simulink model "VDCHyd2022a"  (R2022a)
settings: Solver=daessc  StartTime=0.0  StopTime=simulationEndTime  FixedStep=0.001  RelTol=1e-2
values from neighbouring files (symbols this model uses):
  aux = thetaXrLB(i)    [initInertiaUpdate.m]
  Bc1_V = [0;0;0;0;0;0]    [InitializeSimulationParameters.m]
  Bc1_Vr = [0;0;0;0;0;0]    [InitializeSimulationParameters.m]
  D22Fr = [0;0;0;0;0;0]    [InitializeSimulationParameters.m]
  filtDF = init2ndOrderLowPassFilter(filtDF.cutOffFrequency,1,controller.dT)    [initializeLowPassFilters.m]
  filtDV = init2ndOrderLowPassFilter(filtDV.cutOffFrequency,1,controller.dT)    [initializeLowPassFilters.m]
  filtEnc = init2ndOrderLowPassFilter(filtEnc.cutOffFrequency,1,controller.dT)    [initializeLowPassFilters.m]
  filtPres = init2ndOrderLowPassFilter(filtPres.cutOffFrequency,1,controller.dT)    [initializeLowPassFilters.m]
  MODE = 1    [RUN_ME.m]
  s = tf('s')    [init2ndOrderLowPassFilter.m]
undefined symbols (not defined in the file or in its folder): B11_r_B11Tc1, B11_V, B11_Vr, B11Ftot_r, B12_r_B12Tc2, B12_Rot_Tc2, B12_U_Tc2, B12_V, B12_Vr, B12Ftot_r, B31_r_B31B41, B31_V, B31_Vr, B31FTot_r, B32_r_B32B42, B32_Rot_B42, B32_U_B42, B32_V, B32_Vr, B32FTot_r, B41_r_B41Tc1, B41_V, B41_Vr, B41FTot_r, B42_r_B42Tc2, B42_Rot_Tc2, B42_U_Tc2, B42_V, B42_Vr, B42FTot_r, B52_r_B52P32, B52_Rot_P32, B52_U_P32, B52_V, B52_Vr, B52Ftot_r, Bc1_r_Bc1B11, Bc1_r_Bc1B31, Bc1FTot_r, Bc2_r_Bc2B12, Bc2_r_Bc2B32, Bc2_Rot_B12, Bc2_Rot_B32, Bc2_U_B12, Bc2_U_B32, Bc2_V, Bc2_Vr, Bc2Tot_r, controller, cyl1, cyl2, cylT2, D22_V, D22_Vr, DiscIntNeverNeededParam, dq1, dq11, dq11r, dq12, dq12r ... (+119)
libraries: sm_lib x34, nesl_utility x15, simulink x11, dspinverses x1
(part 10 of 12)

== system VDCHyd2022a/sbVDCController/sbFormTotalRequiredForces/sbTotalRequiredForcesRS2/sbFilteredVelocityDerivativeB32/sbLowPassFilter6 ==
  dV : Inport
  Delay : Delay  InitialConditionSource=Input port  SampleTime=filtDV.dT
      settings: InputPortMap=u0,p4
  Delay1 : Delay  DelayLength=1  InitialConditionSource=Input port  SampleTime=filtDV.dT
      settings: InputPortMap=u0,p4
  Delay2 : Delay  DelayLength=0  InitialConditionSource=Input port  SampleTime=filtDV.dT
      settings: InputPortMap=u0,p4
  Delay3 : Delay  InitialConditionSource=Input port  SampleTime=filtDV.dT
      settings: InputPortMap=u0,p4
  Delay4 : Delay  DelayLength=1  InitialConditionSource=Input port  SampleTime=filtDV.dT
      settings: InputPortMap=u0,p4
  Gain : Gain  Gain=filtDV.a0
  Gain1 : Gain  Gain=filtDV.b1
  Gain2 : Gain  Gain=filtDV.b2
  Gain3 : Gain  Gain=filtDV.b0
  Gain4 : Gain  Gain=filtDV.a1
  Sum : Sum  Inputs=|--+++
  dVFilt : Outport
  wires:
  Delay3/1 -> Gain3/1
  Gain/1 -> Sum/2
  Gain1/1 -> Sum/4
  dV/1 -> Delay/2, Delay4/2, Delay1/2, Delay3/1, Delay3/2, Delay1/1, Delay2/2, Delay2/1  "dV"
  Sum/1 -> Delay/1, Delay4/1, dVFilt/1  "dVFilt"
  Gain4/1 -> Sum/1
  Delay2/1 -> Gain2/1
  Delay1/1 -> Gain1/1
  Delay/1 -> Gain/1
  Delay4/1 -> Gain4/1
  Gain2/1 -> Sum/3
  Gain3/1 -> Sum/5

== system VDCHyd2022a/sbVDCController/sbFormTotalRequiredForces/sbTotalRequiredForcesRS2/sbFilteredVelocityDerivativeB42/sbDiscreteDerivative1 ==
  u : Inport
  Add : Sum  Inputs=-+
  Gain6 : Gain  Gain=1/(2*controller.dT)
  Integer Delay : Delay  InitialConditionSource=Input port  InitialCondition=0  SampleTime=controller.dT
      settings: InputPortMap=u0,p4
  du/dt : Outport  PortDimensions=1
  wires:
  Add/1 -> Gain6/1
  u/1 -> Integer Delay/1, Integer Delay/2, Add/2
  Integer Delay/1 -> Add/1
  Gain6/1 -> du/dt/1

== system VDCHyd2022a/sbVDCController/sbFormTotalRequiredForces/sbTotalRequiredForcesRS2/sbFilteredVelocityDerivativeB42/sbDiscreteDerivative2 ==
  u : Inport
  Add : Sum  Inputs=-+
  Gain6 : Gain  Gain=1/(2*controller.dT)
  Integer Delay : Delay  InitialConditionSource=Input port  InitialCondition=0  SampleTime=controller.dT
      settings: InputPortMap=u0,p4
  du/dt : Outport  PortDimensions=1
  wires:
  u/1 -> Integer Delay/1, Integer Delay/2, Add/2
  Integer Delay/1 -> Add/1
  Add/1 -> Gain6/1
  Gain6/1 -> du/dt/1

== system VDCHyd2022a/sbVDCController/sbFormTotalRequiredForces/sbTotalRequiredForcesRS2/sbFilteredVelocityDerivativeB42/sbDiscreteDerivative3 ==
  u : Inport
  Add : Sum  Inputs=-+
  Gain6 : Gain  Gain=1/(2*controller.dT)
  Integer Delay : Delay  InitialConditionSource=Input port  InitialCondition=0  SampleTime=controller.dT
      settings: InputPortMap=u0,p4
  du/dt : Outport  PortDimensions=1
  wires:
  Add/1 -> Gain6/1
  Integer Delay/1 -> Add/1
  u/1 -> Integer Delay/1, Integer Delay/2, Add/2
  Gain6/1 -> du/dt/1

== system VDCHyd2022a/sbVDCController/sbFormTotalRequiredForces/sbTotalRequiredForcesRS2/sbFilteredVelocityDerivativeB42/sbDiscreteDerivative4 ==
  u : Inport
  Add : Sum  Inputs=-+
  Gain6 : Gain  Gain=1/(2*controller.dT)
  Integer Delay : Delay  InitialConditionSource=Input port  InitialCondition=0  SampleTime=controller.dT
      settings: InputPortMap=u0,p4
  du/dt : Outport  PortDimensions=1
  wires:
  Add/1 -> Gain6/1
  Integer Delay/1 -> Add/1
  u/1 -> Integer Delay/1, Integer Delay/2, Add/2
  Gain6/1 -> du/dt/1

== system VDCHyd2022a/sbVDCController/sbFormTotalRequiredForces/sbTotalRequiredForcesRS2/sbFilteredVelocityDerivativeB42/sbDiscreteDerivative5 ==
  u : Inport
  Add : Sum  Inputs=-+
  Gain6 : Gain  Gain=1/(2*controller.dT)
  Integer Delay : Delay  InitialConditionSource=Input port  InitialCondition=0  SampleTime=controller.dT
      settings: InputPortMap=u0,p4
  du/dt : Outport  PortDimensions=1
  wires:
  Add/1 -> Gain6/1
  Integer Delay/1 -> Add/1
  u/1 -> Integer Delay/1, Integer Delay/2, Add/2
  Gain6/1 -> du/dt/1

== system VDCHyd2022a/sbVDCController/sbFormTotalRequiredForces/sbTotalRequiredForcesRS2/sbFilteredVelocityDerivativeB42/sbDiscreteDerivative6 ==
  u : Inport
  Add : Sum  Inputs=-+
  Gain6 : Gain  Gain=1/(2*controller.dT)
  Integer Delay : Delay  InitialConditionSource=Input port  InitialCondition=0  SampleTime=controller.dT
      settings: InputPortMap=u0,p4
  du/dt : Outport  PortDimensions=1
  wires:
  Add/1 -> Gain6/1
  Integer Delay/1 -> Add/1
  u/1 -> Integer Delay/1, Integer Delay/2, Add/2
  Gain6/1 -> du/dt/1

== system VDCHyd2022a/sbVDCController/sbFormTotalRequiredForces/sbTotalRequiredForcesRS2/sbFilteredVelocityDerivativeB42/sbLowPassFilter1 ==
  dV : Inport
  Delay : Delay  InitialConditionSource=Input port  SampleTime=filtDV.dT
      settings: InputPortMap=u0,p4
  Delay1 : Delay  DelayLength=1  InitialConditionSource=Input port  SampleTime=filtDV.dT
      settings: InputPortMap=u0,p4
  Delay2 : Delay  DelayLength=0  InitialConditionSource=Input port  SampleTime=filtDV.dT
      settings: InputPortMap=u0,p4
  Delay3 : Delay  InitialConditionSource=Input port  SampleTime=filtDV.dT
      settings: InputPortMap=u0,p4
  Delay4 : Delay  DelayLength=1  InitialConditionSource=Input port  SampleTime=filtDV.dT
      settings: InputPortMap=u0,p4
  Gain : Gain  Gain=filtDV.a0
  Gain1 : Gain  Gain=filtDV.b1
  Gain2 : Gain  Gain=filtDV.b2
  Gain3 : Gain  Gain=filtDV.b0
  Gain4 : Gain  Gain=filtDV.a1
  Sum : Sum  Inputs=|--+++
  dVFilt : Outport
  wires:
  Gain3/1 -> Sum/5
  Gain2/1 -> Sum/3
  Delay4/1 -> Gain4/1
  Delay/1 -> Gain/1
  Delay1/1 -> Gain1/1
  Delay2/1 -> Gain2/1
  Gain4/1 -> Sum/1
  Sum/1 -> dVFilt/1, Delay4/1, Delay/1  "dVFilt"
  dV/1 -> Delay2/1, Delay2/2, Delay1/1, Delay3/2, Delay3/1, Delay1/2, Delay4/2, Delay/2  "dV"
  Gain1/1 -> Sum/4
  Gain/1 -> Sum/2
  Delay3/1 -> Gain3/1

== system VDCHyd2022a/sbVDCController/sbFormTotalRequiredForces/sbTotalRequiredForcesRS2/sbFilteredVelocityDerivativeB42/sbLowPassFilter2 ==
  dV : Inport
  Delay : Delay  InitialConditionSource=Input port  SampleTime=filtDV.dT
      settings: InputPortMap=u0,p4
  Delay1 : Delay  DelayLength=1  InitialConditionSource=Input port  SampleTime=filtDV.dT
      settings: InputPortMap=u0,p4
  Delay2 : Delay  DelayLength=0  InitialConditionSource=Input port  SampleTime=filtDV.dT
      settings: InputPortMap=u0,p4
  Delay3 : Delay  InitialConditionSource=Input port  SampleTime=filtDV.dT
      settings: InputPortMap=u0,p4
  Delay4 : Delay  DelayLength=1  InitialConditionSource=Input port  SampleTime=filtDV.dT
      settings: InputPortMap=u0,p4
  Gain : Gain  Gain=filtDV.a0
  Gain1 : Gain  Gain=filtDV.b1
  Gain2 : Gain  Gain=filtDV.b2
  Gain3 : Gain  Gain=filtDV.b0
  Gain4 : Gain  Gain=filtDV.a1
  Sum : Sum  Inputs=|--+++
  dVFilt : Outport
  wires:
  Delay3/1 -> Gain3/1
  Gain/1 -> Sum/2
  Gain1/1 -> Sum/4
  dV/1 -> Delay/2, Delay4/2, Delay1/2, Delay3/1, Delay3/2, Delay1/1, Delay2/2, Delay2/1  "dV"
  Sum/1 -> Delay/1, Delay4/1, dVFilt/1  "dVFilt"
  Gain4/1 -> Sum/1
  Delay2/1 -> Gain2/1
  Delay1/1 -> Gain1/1
  Delay/1 -> Gain/1
  Delay4/1 -> Gain4/1
  Gain2/1 -> Sum/3
  Gain3/1 -> Sum/5

== system VDCHyd2022a/sbVDCController/sbFormTotalRequiredForces/sbTotalRequiredForcesRS2/sbFilteredVelocityDerivativeB42/sbLowPassFilter3 ==
  dV : Inport
  Delay : Delay  InitialConditionSource=Input port  SampleTime=filtDV.dT
      settings: InputPortMap=u0,p4
  Delay1 : Delay  DelayLength=1  InitialConditionSource=Input port  SampleTime=filtDV.dT
      settings: InputPortMap=u0,p4
  Delay2 : Delay  DelayLength=0  InitialConditionSource=Input port  SampleTime=filtDV.dT
      settings: InputPortMap=u0,p4
  Delay3 : Delay  InitialConditionSource=Input port  SampleTime=filtDV.dT
      settings: InputPortMap=u0,p4
  Delay4 : Delay  DelayLength=1  InitialConditionSource=Input port  SampleTime=filtDV.dT
      settings: InputPortMap=u0,p4
  Gain : Gain  Gain=filtDV.a0
  Gain1 : Gain  Gain=filtDV.b1
  Gain2 : Gain  Gain=filtDV.b2
  Gain3 : Gain  Gain=filtDV.b0
  Gain4 : Gain  Gain=filtDV.a1
  Sum : Sum  Inputs=|--+++
  dVFilt : Outport
  wires:
  Gain3/1 -> Sum/5
  Gain2/1 -> Sum/3
  Delay4/1 -> Gain4/1
  Delay/1 -> Gain/1
  Delay1/1 -> Gain1/1
  Delay2/1 -> Gain2/1
  Gain4/1 -> Sum/1
  Sum/1 -> dVFilt/1, Delay4/1, Delay/1  "dVFilt"
  dV/1 -> Delay2/1, Delay2/2, Delay1/1, Delay3/2, Delay3/1, Delay1/2, Delay4/2, Delay/2  "dV"
  Gain1/1 -> Sum/4
  Gain/1 -> Sum/2
  Delay3/1 -> Gain3/1

== system VDCHyd2022a/sbVDCController/sbFormTotalRequiredForces/sbTotalRequiredForcesRS2/sbFilteredVelocityDerivativeB42/sbLowPassFilter4 ==
  dV : Inport
  Delay : Delay  InitialConditionSource=Input port  SampleTime=filtDV.dT
      settings: InputPortMap=u0,p4
  Delay1 : Delay  DelayLength=1  InitialConditionSource=Input port  SampleTime=filtDV.dT
      settings: InputPortMap=u0,p4
  Delay2 : Delay  DelayLength=0  InitialConditionSource=Input port  SampleTime=filtDV.dT
      settings: InputPortMap=u0,p4
  Delay3 : Delay  InitialConditionSource=Input port  SampleTime=filtDV.dT
      settings: InputPortMap=u0,p4
  Delay4 : Delay  DelayLength=1  InitialConditionSource=Input port  SampleTime=filtDV.dT
      settings: InputPortMap=u0,p4
  Gain : Gain  Gain=filtDV.a0
  Gain1 : Gain  Gain=filtDV.b1
  Gain2 : Gain  Gain=filtDV.b2
  Gain3 : Gain  Gain=filtDV.b0
  Gain4 : Gain  Gain=filtDV.a1
  Sum : Sum  Inputs=|--+++
  dVFilt : Outport
  wires:
  Delay3/1 -> Gain3/1
  Gain/1 -> Sum/2
  Gain1/1 -> Sum/4
  dV/1 -> Delay/2, Delay4/2, Delay1/2, Delay3/1, Delay3/2, Delay1/1, Delay2/2, Delay2/1  "dV"
  Sum/1 -> Delay/1, Delay4/1, dVFilt/1  "dVFilt"
  Gain4/1 -> Sum/1
  Delay2/1 -> Gain2/1
  Delay1/1 -> Gain1/1
  Delay/1 -> Gain/1
  Delay4/1 -> Gain4/1
  Gain2/1 -> Sum/3
  Gain3/1 -> Sum/5

== system VDCHyd2022a/sbVDCController/sbFormTotalRequiredForces/sbTotalRequiredForcesRS2/sbFilteredVelocityDerivativeB42/sbLowPassFilter5 ==
  dV : Inport
  Delay : Delay  InitialConditionSource=Input port  SampleTime=filtDV.dT
      settings: InputPortMap=u0,p4
  Delay1 : Delay  DelayLength=1  InitialConditionSource=Input port  SampleTime=filtDV.dT
      settings: InputPortMap=u0,p4
  Delay2 : Delay  DelayLength=0  InitialConditionSource=Input port  SampleTime=filtDV.dT
      settings: InputPortMap=u0,p4
  Delay3 : Delay  InitialConditionSource=Input port  SampleTime=filtDV.dT
      settings: InputPortMap=u0,p4
  Delay4 : Delay  DelayLength=1  InitialConditionSource=Input port  SampleTime=filtDV.dT
      settings: InputPortMap=u0,p4
  Gain : Gain  Gain=filtDV.a0
  Gain1 : Gain  Gain=filtDV.b1
  Gain2 : Gain  Gain=filtDV.b2
  Gain3 : Gain  Gain=filtDV.b0
  Gain4 : Gain  Gain=filtDV.a1
  Sum : Sum  Inputs=|--+++
  dVFilt : Outport
  wires:
  Gain3/1 -> Sum/5
  Gain2/1 -> Sum/3
  Delay4/1 -> Gain4/1
  Delay/1 -> Gain/1
  Delay1/1 -> Gain1/1
  Delay2/1 -> Gain2/1
  Gain4/1 -> Sum/1
  Sum/1 -> dVFilt/1, Delay4/1, Delay/1  "dVFilt"
  dV/1 -> Delay2/1, Delay2/2, Delay1/1, Delay3/2, Delay3/1, Delay1/2, Delay4/2, Delay/2  "dV"
  Gain1/1 -> Sum/4
  Gain/1 -> Sum/2
  Delay3/1 -> Gain3/1

== system VDCHyd2022a/sbVDCController/sbFormTotalRequiredForces/sbTotalRequiredForcesRS2/sbFilteredVelocityDerivativeB42/sbLowPassFilter6 ==
  dV : Inport
  Delay : Delay  InitialConditionSource=Input port  SampleTime=filtDV.dT
      settings: InputPortMap=u0,p4
  Delay1 : Delay  DelayLength=1  InitialConditionSource=Input port  SampleTime=filtDV.dT
      settings: InputPortMap=u0,p4
  Delay2 : Delay  DelayLength=0  InitialConditionSource=Input port  SampleTime=filtDV.dT
      settings: InputPortMap=u0,p4
  Delay3 : Delay  InitialConditionSource=Input port  SampleTime=filtDV.dT
      settings: InputPortMap=u0,p4
  Delay4 : Delay  DelayLength=1  InitialConditionSource=Input port  SampleTime=filtDV.dT
      settings: InputPortMap=u0,p4
  Gain : Gain  Gain=filtDV.a0
  Gain1 : Gain  Gain=filtDV.b1
  Gain2 : Gain  Gain=filtDV.b2
  Gain3 : Gain  Gain=filtDV.b0
  Gain4 : Gain  Gain=filtDV.a1
  Sum : Sum  Inputs=|--+++
  dVFilt : Outport
  wires:
  Delay3/1 -> Gain3/1
  Gain/1 -> Sum/2
  Gain1/1 -> Sum/4
  dV/1 -> Delay/2, Delay4/2, Delay1/2, Delay3/1, Delay3/2, Delay1/1, Delay2/2, Delay2/1  "dV"
  Sum/1 -> Delay/1, Delay4/1, dVFilt/1  "dVFilt"
  Gain4/1 -> Sum/1
  Delay2/1 -> Gain2/1
  Delay1/1 -> Gain1/1
  Delay/1 -> Gain/1
  Delay4/1 -> Gain4/1
  Gain2/1 -> Sum/3
  Gain3/1 -> Sum/5

== system VDCHyd2022a/sbVDCController/sbFormTotalRequiredForces/sbTotalRequiredForcesRS2/sbFilteredVelocityDerivativeBc2/sbDiscreteDerivative1 ==
  u : Inport
  Add : Sum  Inputs=-+
  Gain6 : Gain  Gain=1/(2*controller.dT)
  Integer Delay : Delay  InitialConditionSource=Input port  InitialCondition=0  SampleTime=controller.dT
      settings: InputPortMap=u0,p4
  du/dt : Outport  PortDimensions=1
  wires:
  Add/1 -> Gain6/1
  u/1 -> Integer Delay/1, Integer Delay/2, Add/2
  Integer Delay/1 -> Add/1
  Gain6/1 -> du/dt/1

== system VDCHyd2022a/sbVDCController/sbFormTotalRequiredForces/sbTotalRequiredForcesRS2/sbFilteredVelocityDerivativeBc2/sbDiscreteDerivative2 ==
  u : Inport
  Add : Sum  Inputs=-+
  Gain6 : Gain  Gain=1/(2*controller.dT)
  Integer Delay : Delay  InitialConditionSource=Input port  InitialCondition=0  SampleTime=controller.dT
      settings: InputPortMap=u0,p4
  du/dt : Outport  PortDimensions=1
  wires:
  u/1 -> Integer Delay/1, Integer Delay/2, Add/2
  Integer Delay/1 -> Add/1
  Add/1 -> Gain6/1
  Gain6/1 -> du/dt/1

== system VDCHyd2022a/sbVDCController/sbFormTotalRequiredForces/sbTotalRequiredForcesRS2/sbFilteredVelocityDerivativeBc2/sbDiscreteDerivative3 ==
  u : Inport
  Add : Sum  Inputs=-+
  Gain6 : Gain  Gain=1/(2*controller.dT)
  Integer Delay : Delay  InitialConditionSource=Input port  InitialCondition=0  SampleTime=controller.dT
      settings: InputPortMap=u0,p4
  du/dt : Outport  PortDimensions=1
  wires:
  Add/1 -> Gain6/1
  Integer Delay/1 -> Add/1
  u/1 -> Integer Delay/1, Integer Delay/2, Add/2
  Gain6/1 -> du/dt/1

== system VDCHyd2022a/sbVDCController/sbFormTotalRequiredForces/sbTotalRequiredForcesRS2/sbFilteredVelocityDerivativeBc2/sbDiscreteDerivative4 ==
  u : Inport
  Add : Sum  Inputs=-+
  Gain6 : Gain  Gain=1/(2*controller.dT)
  Integer Delay : Delay  InitialConditionSource=Input port  InitialCondition=0  SampleTime=controller.dT
      settings: InputPortMap=u0,p4
  du/dt : Outport  PortDimensions=1
  wires:
  Add/1 -> Gain6/1
  Integer Delay/1 -> Add/1
  u/1 -> Integer Delay/1, Integer Delay/2, Add/2
  Gain6/1 -> du/dt/1

== system VDCHyd2022a/sbVDCController/sbFormTotalRequiredForces/sbTotalRequiredForcesRS2/sbFilteredVelocityDerivativeBc2/sbDiscreteDerivative5 ==
  u : Inport
  Add : Sum  Inputs=-+
  Gain6 : Gain  Gain=1/(2*controller.dT)
  Integer Delay : Delay  InitialConditionSource=Input port  InitialCondition=0  SampleTime=controller.dT
      settings: InputPortMap=u0,p4
  du/dt : Outport  PortDimensions=1
  wires:
  Add/1 -> Gain6/1
  Integer Delay/1 -> Add/1
  u/1 -> Integer Delay/1, Integer Delay/2, Add/2
  Gain6/1 -> du/dt/1

== system VDCHyd2022a/sbVDCController/sbFormTotalRequiredForces/sbTotalRequiredForcesRS2/sbFilteredVelocityDerivativeBc2/sbDiscreteDerivative6 ==
  u : Inport
  Add : Sum  Inputs=-+
  Gain6 : Gain  Gain=1/(2*controller.dT)
  Integer Delay : Delay  InitialConditionSource=Input port  InitialCondition=0  SampleTime=controller.dT
      settings: InputPortMap=u0,p4
  du/dt : Outport  PortDimensions=1
  wires:
  Add/1 -> Gain6/1
  Integer Delay/1 -> Add/1
  u/1 -> Integer Delay/1, Integer Delay/2, Add/2
  Gain6/1 -> du/dt/1

== system VDCHyd2022a/sbVDCController/sbFormTotalRequiredForces/sbTotalRequiredForcesRS2/sbFilteredVelocityDerivativeBc2/sbLowPassFilter1 ==
  dV : Inport
  Delay : Delay  InitialConditionSource=Input port  SampleTime=filtDV.dT
      settings: InputPortMap=u0,p4
  Delay1 : Delay  DelayLength=1  InitialConditionSource=Input port  SampleTime=filtDV.dT
      settings: InputPortMap=u0,p4
  Delay2 : Delay  DelayLength=0  InitialConditionSource=Input port  SampleTime=filtDV.dT
      settings: InputPortMap=u0,p4
  Delay3 : Delay  InitialConditionSource=Input port  SampleTime=filtDV.dT
      settings: InputPortMap=u0,p4
  Delay4 : Delay  DelayLength=1  InitialConditionSource=Input port  SampleTime=filtDV.dT
      settings: InputPortMap=u0,p4
  Gain : Gain  Gain=filtDV.a0
  Gain1 : Gain  Gain=filtDV.b1
  Gain2 : Gain  Gain=filtDV.b2
  Gain3 : Gain  Gain=filtDV.b0
  Gain4 : Gain  Gain=filtDV.a1
  Sum : Sum  Inputs=|--+++
  dVFilt : Outport
  wires:
  Gain3/1 -> Sum/5
  Gain2/1 -> Sum/3
  Delay4/1 -> Gain4/1
  Delay/1 -> Gain/1
  Delay1/1 -> Gain1/1
  Delay2/1 -> Gain2/1
  Gain4/1 -> Sum/1
  Sum/1 -> dVFilt/1, Delay4/1, Delay/1  "dVFilt"
  dV/1 -> Delay2/1, Delay2/2, Delay1/1, Delay3/2, Delay3/1, Delay1/2, Delay4/2, Delay/2  "dV"
  Gain1/1 -> Sum/4
  Gain/1 -> Sum/2
  Delay3/1 -> Gain3/1

== system VDCHyd2022a/sbVDCController/sbFormTotalRequiredForces/sbTotalRequiredForcesRS2/sbFilteredVelocityDerivativeBc2/sbLowPassFilter2 ==
  dV : Inport
  Delay : Delay  InitialConditionSource=Input port  SampleTime=filtDV.dT
      settings: InputPortMap=u0,p4
  Delay1 : Delay  DelayLength=1  InitialConditionSource=Input port  SampleTime=filtDV.dT
      settings: InputPortMap=u0,p4
  Delay2 : Delay  DelayLength=0  InitialConditionSource=Input port  SampleTime=filtDV.dT
      settings: InputPortMap=u0,p4
  Delay3 : Delay  InitialConditionSource=Input port  SampleTime=filtDV.dT
      settings: InputPortMap=u0,p4
  Delay4 : Delay  DelayLength=1  InitialConditionSource=Input port  SampleTime=filtDV.dT
      settings: InputPortMap=u0,p4
  Gain : Gain  Gain=filtDV.a0
  Gain1 : Gain  Gain=filtDV.b1
  Gain2 : Gain  Gain=filtDV.b2
  Gain3 : Gain  Gain=filtDV.b0
  Gain4 : Gain  Gain=filtDV.a1
  Sum : Sum  Inputs=|--+++
  dVFilt : Outport
  wires:
  Delay3/1 -> Gain3/1
  Gain/1 -> Sum/2
  Gain1/1 -> Sum/4
  dV/1 -> Delay/2, Delay4/2, Delay1/2, Delay3/1, Delay3/2, Delay1/1, Delay2/2, Delay2/1  "dV"
  Sum/1 -> Delay/1, Delay4/1, dVFilt/1  "dVFilt"
  Gain4/1 -> Sum/1
  Delay2/1 -> Gain2/1
  Delay1/1 -> Gain1/1
  Delay/1 -> Gain/1
  Delay4/1 -> Gain4/1
  Gain2/1 -> Sum/3
  Gain3/1 -> Sum/5

== system VDCHyd2022a/sbVDCController/sbFormTotalRequiredForces/sbTotalRequiredForcesRS2/sbFilteredVelocityDerivativeBc2/sbLowPassFilter3 ==
  dV : Inport
  Delay : Delay  InitialConditionSource=Input port  SampleTime=filtDV.dT
      settings: InputPortMap=u0,p4
  Delay1 : Delay  DelayLength=1  InitialConditionSource=Input port  SampleTime=filtDV.dT
      settings: InputPortMap=u0,p4
  Delay2 : Delay  DelayLength=0  InitialConditionSource=Input port  SampleTime=filtDV.dT
      settings: InputPortMap=u0,p4
  Delay3 : Delay  InitialConditionSource=Input port  SampleTime=filtDV.dT
      settings: InputPortMap=u0,p4
  Delay4 : Delay  DelayLength=1  InitialConditionSource=Input port  SampleTime=filtDV.dT
      settings: InputPortMap=u0,p4
  Gain : Gain  Gain=filtDV.a0
  Gain1 : Gain  Gain=filtDV.b1
  Gain2 : Gain  Gain=filtDV.b2
  Gain3 : Gain  Gain=filtDV.b0
  Gain4 : Gain  Gain=filtDV.a1
  Sum : Sum  Inputs=|--+++
  dVFilt : Outport
  wires:
  Gain3/1 -> Sum/5
  Gain2/1 -> Sum/3
  Delay4/1 -> Gain4/1
  Delay/1 -> Gain/1
  Delay1/1 -> Gain1/1
  Delay2/1 -> Gain2/1
  Gain4/1 -> Sum/1
  Sum/1 -> dVFilt/1, Delay4/1, Delay/1  "dVFilt"
  dV/1 -> Delay2/1, Delay2/2, Delay1/1, Delay3/2, Delay3/1, Delay1/2, Delay4/2, Delay/2  "dV"
  Gain1/1 -> Sum/4
  Gain/1 -> Sum/2
  Delay3/1 -> Gain3/1

== system VDCHyd2022a/sbVDCController/sbFormTotalRequiredForces/sbTotalRequiredForcesRS2/sbFilteredVelocityDerivativeBc2/sbLowPassFilter4 ==
  dV : Inport
  Delay : Delay  InitialConditionSource=Input port  SampleTime=filtDV.dT
      settings: InputPortMap=u0,p4
  Delay1 : Delay  DelayLength=1  InitialConditionSource=Input port  SampleTime=filtDV.dT
      settings: InputPortMap=u0,p4
  Delay2 : Delay  DelayLength=0  InitialConditionSource=Input port  SampleTime=filtDV.dT
      settings: InputPortMap=u0,p4
  Delay3 : Delay  InitialConditionSource=Input port  SampleTime=filtDV.dT
      settings: InputPortMap=u0,p4
  Delay4 : Delay  DelayLength=1  InitialConditionSource=Input port  SampleTime=filtDV.dT
      settings: InputPortMap=u0,p4
  Gain : Gain  Gain=filtDV.a0
  Gain1 : Gain  Gain=filtDV.b1
  Gain2 : Gain  Gain=filtDV.b2
  Gain3 : Gain  Gain=filtDV.b0
  Gain4 : Gain  Gain=filtDV.a1
  Sum : Sum  Inputs=|--+++
  dVFilt : Outport
  wires:
  Delay3/1 -> Gain3/1
  Gain/1 -> Sum/2
  Gain1/1 -> Sum/4
  dV/1 -> Delay/2, Delay4/2, Delay1/2, Delay3/1, Delay3/2, Delay1/1, Delay2/2, Delay2/1  "dV"
  Sum/1 -> Delay/1, Delay4/1, dVFilt/1  "dVFilt"
  Gain4/1 -> Sum/1
  Delay2/1 -> Gain2/1
  Delay1/1 -> Gain1/1
  Delay/1 -> Gain/1
  Delay4/1 -> Gain4/1
  Gain2/1 -> Sum/3
  Gain3/1 -> Sum/5

== system VDCHyd2022a/sbVDCController/sbFormTotalRequiredForces/sbTotalRequiredForcesRS2/sbFilteredVelocityDerivativeBc2/sbLowPassFilter5 ==
  dV : Inport
  Delay : Delay  InitialConditionSource=Input port  SampleTime=filtDV.dT
      settings: InputPortMap=u0,p4
  Delay1 : Delay  DelayLength=1  InitialConditionSource=Input port  SampleTime=filtDV.dT
      settings: InputPortMap=u0,p4
  Delay2 : Delay  DelayLength=0  InitialConditionSource=Input port  SampleTime=filtDV.dT
      settings: InputPortMap=u0,p4
  Delay3 : Delay  InitialConditionSource=Input port  SampleTime=filtDV.dT
      settings: InputPortMap=u0,p4
  Delay4 : Delay  DelayLength=1  InitialConditionSource=Input port  SampleTime=filtDV.dT
      settings: InputPortMap=u0,p4
  Gain : Gain  Gain=filtDV.a0
  Gain1 : Gain  Gain=filtDV.b1
  Gain2 : Gain  Gain=filtDV.b2
  Gain3 : Gain  Gain=filtDV.b0
  Gain4 : Gain  Gain=filtDV.a1
  Sum : Sum  Inputs=|--+++
  dVFilt : Outport
  wires:
  Gain3/1 -> Sum/5
  Gain2/1 -> Sum/3
  Delay4/1 -> Gain4/1
  Delay/1 -> Gain/1
  Delay1/1 -> Gain1/1
  Delay2/1 -> Gain2/1
  Gain4/1 -> Sum/1
  Sum/1 -> dVFilt/1, Delay4/1, Delay/1  "dVFilt"
  dV/1 -> Delay2/1, Delay2/2, Delay1/1, Delay3/2, Delay3/1, Delay1/2, Delay4/2, Delay/2  "dV"
  Gain1/1 -> Sum/4
  Gain/1 -> Sum/2
  Delay3/1 -> Gain3/1

== system VDCHyd2022a/sbVDCController/sbFormTotalRequiredForces/sbTotalRequiredForcesRS2/sbFilteredVelocityDerivativeBc2/sbLowPassFilter6 ==
  dV : Inport
  Delay : Delay  InitialConditionSource=Input port  SampleTime=filtDV.dT
      settings: InputPortMap=u0,p4
  Delay1 : Delay  DelayLength=1  InitialConditionSource=Input port  SampleTime=filtDV.dT
      settings: InputPortMap=u0,p4
  Delay2 : Delay  DelayLength=0  InitialConditionSource=Input port  SampleTime=filtDV.dT
      settings: InputPortMap=u0,p4
  Delay3 : Delay  InitialConditionSource=Input port  SampleTime=filtDV.dT
      settings: InputPortMap=u0,p4
  Delay4 : Delay  DelayLength=1  InitialConditionSource=Input port  SampleTime=filtDV.dT
      settings: InputPortMap=u0,p4
  Gain : Gain  Gain=filtDV.a0
  Gain1 : Gain  Gain=filtDV.b1
  Gain2 : Gain  Gain=filtDV.b2
  Gain3 : Gain  Gain=filtDV.b0
  Gain4 : Gain  Gain=filtDV.a1
  Sum : Sum  Inputs=|--+++
  dVFilt : Outport
  wires:
  Delay3/1 -> Gain3/1
  Gain/1 -> Sum/2
  Gain1/1 -> Sum/4
  dV/1 -> Delay/2, Delay4/2, Delay1/2, Delay3/1, Delay3/2, Delay1/1, Delay2/2, Delay2/1  "dV"
  Sum/1 -> Delay/1, Delay4/1, dVFilt/1  "dVFilt"
  Gain4/1 -> Sum/1
  Delay2/1 -> Gain2/1
  Delay1/1 -> Gain1/1
  Delay/1 -> Gain/1
  Delay4/1 -> Gain4/1
  Gain2/1 -> Sum/3
  Gain3/1 -> Sum/5

== system VDCHyd2022a/sbVDCController/sbFormAnalyticQuantities/sbRevoluteSegment1/sbGeomPropRS1/sbq1AngleRate/sbDiscreteDerivative ==
  note: Overview of different differentiation scheme can be found in:
      | Harrison, A. J. L., and D. P. Stoten. "Generalized finite difference methods for optimal estimation of derivatives in real-time control problems." Proceedings of the institution of mechanical engineers, part I: journal of systems and control engineering 209.2 (1995): 67-78.
  q1Angle : Inport
  Add : Sum  Inputs=-+
  Gain6 : Gain  Gain=1/(2*controller.dT)
  Integer Delay : Delay  InitialConditionSource=Input port  InitialCondition=0  SampleTime=controller.dT
      settings: InputPortMap=u0,p4
  q1AngleRate : Outport  PortDimensions=1
  wires:
  q1Angle/1 -> Integer Delay/1, Integer Delay/2, Add/2
  Gain6/1 -> q1AngleRate/1
  Integer Delay/1 -> Add/1
  Add/1 -> Gain6/1

== system VDCHyd2022a/sbVDCController/sbFormAnalyticQuantities/sbRevoluteSegment2/sbGeomPropRS2/sbq2AngleRate/sbDiscreteDerivative ==
  q2Angle : Inport
  Add : Sum  Inputs=-+
  Gain6 : Gain  Gain=1/(2*controller.dT)
  Integer Delay : Delay  InitialConditionSource=Input port  InitialCondition=0  SampleTime=controller.dT
      settings: InputPortMap=u0,p4
  q2AngleRate : Outport  PortDimensions=1
  wires:
  q2Angle/1 -> Integer Delay/1, Integer Delay/2, Add/2
  Gain6/1 -> q2AngleRate/1
  Integer Delay/1 -> Add/1
  Add/1 -> Gain6/1

== matlab function VDCHyd2022a/sbVDCController/sbFormAnalyticQuantities/sbRevoluteSegment1/sbGeomPropRS1/sbLiftPistonStroke/liftPistonStroke ==
  data: q1 input; x1 output; geom parameter; cyl1 parameter
function x1 = liftPistonStroke(q1, geom, cyl1)

    % Calculates lift piston stroke per the paper equation (18).
    x1 = sqrt(geom.L1*geom.L1+geom.L11*geom.L11+2*geom.L1*geom.L11*cos(q1))-cyl1.x0;

end

== matlab function VDCHyd2022a/sbVDCController/sbFormAnalyticQuantities/sbRevoluteSegment1/sbGeomPropRS1/sbq11AngleValue/q11AngleValue ==
  data: x1 input; q11 output; geom parameter; cyl1 parameter
function q11 = q11AngleValue(x1, geom, cyl1)

    % Calculates q11-angle per the paper equation (19).
    q11 = -acos((geom.L11*geom.L11-(x1+cyl1.x0)*(x1+cyl1.x0)-geom.L1*geom.L1)/(-2*(x1+cyl1.x0)*geom.L1));

end

== matlab function VDCHyd2022a/sbVDCController/sbAuxiliaryJointAngles/q1Angle ==
  data: theta1 input; q1 output; geom parameter
function q1 = q1Angle(theta1, geom)

    % Calculates q1 angle value from the encoder- (or other by means-)
    % obtained angle theta1. 
    q1 = -pi/2 - geom.beta1 - geom.beta2 + theta1;

end

== matlab function VDCHyd2022a/sbVDCController/sbAuxiliaryJointAngles/q2Angle ==
  data: theta2 input; q2 output; geom parameter
function q2 = q2Angle(theta2, geom)

    % Calculates q2 angle value from the encoder- (or other by means-)
    % obtained angle Theta2.
    q2 = theta2 - geom.beta3 - geom.beta4;

end

== matlab function VDCHyd2022a/sbHydraulicElements/sbValveFlowsPS1/extensionValveFlows ==
  data: pat2 input; Qat2 output; pbt2 input; ut2v input; pS input; pR input; Qbt2 output; valveT2 parameter
function [Qat2, Qbt2] = extensionValveFlows(pat2, pbt2, ut2v, pS, pR, valveT2)

    % Calculates extension valve flows per the paper equations (82) and (83).
    Qat2 = valveT2.cp1*sqAbsPresDrop(pS - pat2)*ut2v*selFcn(ut2v) + ...
       valveT2.cn1*sqAbsPresDrop(pat2 - pR)*ut2v*selFcn(-ut2v);
    Qbt2 = -valveT2.cn2*sqAbsPresDrop(pbt2 - pR)*ut2v*selFcn(ut2v) - ...
       valveT2.cp2*sqAbsPresDrop(pS - pbt2)*ut2v*selFcn(-ut2v);
   
end

function S = selFcn(U)

    % Implements the selection function (84). 
    if U > 0
        S = 1;
    else
        S = 0;
    end
    
end

function nup = sqAbsPresDrop(dp)

    % Implements the pressure drop function (85).
    nup = sign(dp)*sqrt(abs(dp));

end

== matlab function VDCHyd2022a/sbVDCController/sbFormAnalyticQuantities/sbRevoluteSegment1/sbGeomPropRS1/sbq12AngleValue/q12AngleValue ==
  data: x1 input; q12 output; geom parameter; cyl1 parameter
function q12 = q12AngleValue(x1, geom, cyl1)

    % Calculates q12-angle per the paper equation (20).
    q12 = -acos((geom.L1*geom.L1-(x1+cyl1.x0)*(x1+cyl1.x0)-geom.L11*geom.L11)/(-2*(x1+cyl1.x0)*geom.L11));

end

== matlab function VDCHyd2022a/sbVDCController/sbFormAnalyticQuantities/sbRevoluteSegment2/sbGeomPropRS2/sbq21AngleValue/q21AngleValue ==
  data: x2 input; q21 output; geom parameter; cyl2 parameter
function q21 = q21AngleValue(x2, geom, cyl2)

    % Calculates q21-angle per the paper equation (19).
    q21 = -acos((geom.L21*geom.L21-(x2+cyl2.x0)*(x2+cyl2.x0)-geom.L2*geom.L2)/(-2*(x2+cyl2.x0)*geom.L2));

end

== matlab function VDCHyd2022a/sbVDCController/sbFormAnalyticQuantities/sbRevoluteSegment2/sbGeomPropRS2/sbq21AngleRate/q21AngleRate ==
  data: x2 input; q21 input; dx2 input; dq21 output; geom parameter; cyl2 parameter
function dq21 = q21AngleRate(x2, q21, dx2, geom, cyl2)
    
    % Calculates q21 angle rate per the paper equation (22).
    dq21 = -((x2+cyl2.x0)-geom.L2*cos(q21))/((x2+cyl2.x0)*geom.L2*sin(q21))*dx2;

end

== matlab function VDCHyd2022a/sbVDCController/sbFormAnalyticQuantities/sbRevoluteSegment2/sbGeomPropRS2/sbTiltPistonVelocity/tiltPistonVelocity ==
  data: dq2 input; x2 input; q2 input; dx2 output; geom parameter; cyl2 parameter
function dx2 = tiltPistonVelocity(dq2, x2, q2, geom, cyl2)

    % Calculates lift piston velocity per the paper equation (21).
    dx2 = -(geom.L2*geom.L21*sin(q2))/(x2+cyl2.x0)*dq2;

end

== matlab function VDCHyd2022a/sbVDCController/sbFormAnalyticQuantities/sbRevoluteSegment2/sbGeomPropRS2/sbq22AngleValue/q22AngleValue ==
  data: x2 input; q22 output; geom parameter; cyl2 parameter
function q22 = q22AngleValue(x2, geom, cyl2)

    % Calculates q22-angle per the paper equation (20).
    q22 = -acos((geom.L2*geom.L2-(x2+cyl2.x0)*(x2+cyl2.x0)-geom.L21*geom.L21)/(-2*(x2+cyl2.x0)*geom.L21));

end

== matlab function VDCHyd2022a/sbVDCController/sbFormAnalyticQuantities/sbRevoluteSegment2/sbGeomPropRS2req/sbRequiredq21AngleRate/requiredq21AngleRate ==
  data: x2 input; q21 input; dx2r input; dq21r output; geom parameter; cyl2 parameter
function dq21r = requiredq21AngleRate(x2, q21, dx2r, geom, cyl2)

    % Calculate the required q21 angle rate per the paper equation (22).
    dq21r = -((x2+cyl2.x0)-geom.L2*cos(q21))/((x2+cyl2.x0)*geom.L2*sin(q21))*dx2r;

end

== matlab function VDCHyd2022a/sbVDCController/sbFormAnalyticQuantities/sbRevoluteSegment2/sbGeomPropRS2/sbq22AngleRate/q22AngleRate ==
  data: x2 input; q22 input; dx2 input; dq22 output; geom parameter; cyl2 parameter
function dq22 = q22AngleRate(x2, q22, dx2, geom, cyl2)

    % Calculates q22 angle rate per the paper equation (23). 
    dq22 = -((x2+cyl2.x0)-geom.L21*cos(q22))/((x2+cyl2.x0)*geom.L21*sin(q22))*dx2;

end

== matlab function VDCHyd2022a/sbVDCController/sbFormAnalyticQuantities/sbRevoluteSegment2/sbGeomPropRS2req/sbRequiredq22AngleRate/requiredq22AngleRate ==
  data: x2 input; q22 input; dx2r input; dq22r output; geom parameter; cyl2 parameter
function dq22r = requiredq22AngleRate(x2, q22, dx2r, geom, cyl2)

    % Calculates the required q12 angle rate per the paper equation (23).
    dq22r = -((x2+cyl2.x0)-geom.L21*cos(q22))/((x2+cyl2.x0)*geom.L21*sin(q22))*dx2r;

end

== matlab function VDCHyd2022a/sbVDCController/sbFormAnalyticQuantities/sbRevoluteSegment2/sbGeomPropRS2/sbTiltPistonStroke/tiltPistonStroke ==
  data: q2 input; x2 output; geom parameter; cyl2 parameter
function x2 = tiltPistonStroke(q2, geom, cyl2)

    % Calculates lift piston stroke per the paper equation (18).
    x2 = sqrt(geom.L2*geom.L2+geom.L21*geom.L21+2*geom.L2*geom.L21*cos(q2))-cyl2.x0;

end

== matlab function VDCHyd2022a/sbHydraulicManipulatorSimscape/sbLiftCylinderAndLiftPiston/sbFrictionForceRS1/sbFrictionRegressorRS1/frictionRegressorFunctionRS1 ==
  data: v input; z input; Yf output; L input; Fd input; frictionRS1 parameter
function Yf = frictionRegressor(v,z,L, Fd, frictionRS1)

    % Forms the friction regressor from Zhu, W. H., & Piedboeuf, J. C. 
    % (2005). Adaptive output force tracking control of hydraulic cylinders 
    % with applications to robot manipulators.
    Yf = [(1 - L)*g(z, frictionRS1.zss)*S(z),...
          -(1 - L)*g(-z, frictionRS1.zss)*S(-z),...
          1 - L,...
          (1 - L)*S(v)*phivp(v)*v,...
          (1 - L)*S(-v)*phivn(v)*v,...
          S(Fd)*L*phifp(Fd,frictionRS1.deltap),...
          S(-Fd)*L*phifn(Fd,frictionRS1.deltan)];

end

function S = S(x)

    % Per (2) from Zhu, W. H., & Piedboeuf, J. C. (2005).
    if x > 0
        S = 1;
    else
        S = 0;
    end

end

function g = g(z, zss)

    % Per (5) in Zhu, W. H., & Piedboeuf, J. C. (2005).
    if z >= zss
        g = 1;
    elseif z <= 0
        g = 0;
    else
        g = z/zss;
    end

end

function phifp = phifp(f, deltafp)

    % Per (6) in Zhu, W. H., & Piedboeuf, J. C. (2005).
    phifp = f/(1 + deltafp*abs(f));

end

function phifn = phifn(f, deltafn)

    % Per (6) in Zhu, W. H., & Piedboeuf, J. C. (2005).
    phifn = f/(1 + deltafn*abs(f));

end

function phivp = phivp(v)

    % Chosen as constant. More details on pp. 211 of Zhu, W. H., & 
    % Piedboeuf, J. C. (2005), just above Eq. (71)
    phivp = 5 + 0*v;

end

function phivn = phivn(v)

    % Chosen as constant. More details on pp. 211 of Zhu, W. H., & 
    % Piedboeuf, J. C. (2005), just above Eq. (71)
    phivn = 5 + 0*v;

end

== matlab function VDCHyd2022a/sbVDCController/sbFormAnalyticQuantities/sbRevoluteSegment2/sbGeomPropRS2req/sbRequiredTiltPistonVelocity/requiredTiltPistonVelocity ==
  data: dq2r input; x2 input; q2 input; dx2r output; geom parameter; cyl2 parameter
function dx2r = requiredTiltPistonVelocity(dq2r, x2, q2, geom, cyl2)

    % calculates required lift piston velocity per the paper equation (21).
    dx2r = -(geom.L2*geom.L21*sin(q2))/(x2+cyl2.x0)*dq2r;

end

== matlab function VDCHyd2022a/sbHydraulicManipulatorSimscape/sbTiltCylinderAndTiltPiston/sbFrictionForceRS2/sbFrictionRegressorRS2/frictionRegressorFunctionRS2 ==
  data: v input; z input; Yf output; L input; Fd input; frictionRS2 parameter
function Yf = frictionRegressor(v,z,L, Fd, frictionRS2)

    % Forms the friction regressor from Zhu, W. H., & Piedboeuf, J. C. 
    % (2005). Adaptive output force tracking control of hydraulic cylinders 
    % with applications to robot manipulators.
    Yf = [(1 - L)*g(z, frictionRS2.zss)*S(z),...
          -(1 - L)*g(-z, frictionRS2.zss)*S(-z),...
          1 - L,...
          (1 - L)*S(v)*phivp(v)*v,...
          (1 - L)*S(-v)*phivn(v)*v,...
          S(Fd)*L*phifp(Fd,frictionRS2.deltap),...
          S(-Fd)*L*phifn(Fd,frictionRS2.deltan)];

end

function S = S(x)

    % Per (2) from Zhu, W. H., & Piedboeuf, J. C. (2005).
    if x > 0
        S = 1;
    else
        S = 0;
    end

end

function g = g(z, zss)

    % Per (5) in Zhu, W. H., & Piedboeuf, J. C. (2005).
    if z >= zss
        g = 1;
    elseif z <= 0
        g = 0;
    else
        g = z/zss;
    end

end

function phifp = phifp(f, deltafp)

    % Per (6) in Zhu, W. H., & Piedboeuf, J. C. (2005).
    phifp = f/(1 + deltafp*abs(f));

end

function phifn = phifn(f, deltafn)

    % Per (6) in Zhu, W. H., & Piedboeuf, J. C. (2005).
    phifn = f/(1 + deltafn*abs(f));

end

function phivp = phivp(v)

    % Chosen as constant. More details on pp. 211 of Zhu, W. H., & 
    % Piedboeuf, J. C. (2005), just above Eq. (71)
    phivp = 5 + 0*v;

end

function phivn = phivn(v)

    % Chosen as constant. More details on pp. 211 of Zhu, W. H., & 
    % Piedboeuf, J. C. (2005), just above Eq. (71)
    phivn = 5 + 0*v;

end

== matlab function VDCHyd2022a/sbVDCController/sbFormingControlActions/controlVoltageRS2 ==
  data: uf2r input; pS input; pR input; pa2 input; pb2 input; x2 input; u2 output; thetav2 input; hosing2 parameter; cyl2 parameter
function u2  = calculateControlVoltage(uf2r, pS, pR, pa2, pb2, x2, thetav2, hosing2, cyl2)

    cp1 = thetav2(1); cn1 = thetav2(2); cp2 = thetav2(3); cn2 = thetav2(4);

    % Implemented per (27) in S. Lampinen, J. Koivumäki and J. Mattila, 
    % "Improved Hydraulic Cylinder Model for the Virtual Decomposition 
    % Control Approach," 2019 IEEE International Conference on Cybernetics 
    % and Intelligent Systems (CIS) and IEEE Conference on Robotics, 
    % Automation and Mechatronics (RAM), Bangkok, Thailand, 2019, 
    % pp. 113-118, doi: 10.1109/CIS-RAM47153.2019.9095788 
    u2 = uf2r*selFcn(uf2r)/( (cp1*sqAbsPresDrop(pS-pa2))/(hosing2.V0a/cyl2.Aa + x2) + (cn2*sqAbsPresDrop(pb2-pR))/(hosing2.V0b/cyl2.Ab + cyl2.sp - x2) ) + ...
         uf2r*selFcn(-uf2r)/( (cp2*sqAbsPresDrop(pS-pb2))/(hosing2.V0b/cyl2.Ab + cyl2.sp - x2) + (cn1*sqAbsPresDrop(pa2-pR))/(hosing2.V0a/cyl2.Aa + x2) );


end


function S = selFcn(U)

    if U > 0
        S = 1;
    else
        S = 0;
    end
    
end

function nup = sqAbsPresDrop(dp)

    nup = sign(dp)*sqrt(abs(dp));

end

== matlab function VDCHyd2022a/sbHydraulicManipulatorSimscape/sbPrismaticJointCylinderAndPiston/sbFrictionForcePS2/sbFrictionRegressorPS2/frictionRegressorFunctionPS2 ==
  data: v input; z input; Yf output; L input; Fd input; frictionPS2 parameter
function Yf = frictionRegressor(v,z,L, Fd, frictionPS2)

    % Forms the friction regressor from Zhu, W. H., & Piedboeuf, J. C. 
    % (2005). Adaptive output force tracking control of hydraulic cylinders 
    % with applications to robot manipulators.
    Yf = [(1 - L)*g(z, frictionPS2.zss)*S(z),...
          -(1 - L)*g(-z, frictionPS2.zss)*S(-z),...
          1 - L,...
          (1 - L)*S(v)*phivp(v)*v,...
          (1 - L)*S(-v)*phivn(v)*v,...
          S(Fd)*L*phifp(Fd,frictionPS2.deltap),...
          S(-Fd)*L*phifn(Fd,frictionPS2.deltan)];

end

function S = S(x)

    % Per (2) from Zhu, W. H., & Piedboeuf, J. C. (2005).
    if x > 0
        S = 1;
    else
        S = 0;
    end

end

function g = g(z, zss)

    % Per (5) in Zhu, W. H., & Piedboeuf, J. C. (2005).
    if z >= zss
        g = 1;
    elseif z <= 0
        g = 0;
    else
        g = z/zss;
    end

end

function phifp = phifp(f, deltafp)

    % Per (6) in Zhu, W. H., & Piedboeuf, J. C. (2005).
    phifp = f/(1 + deltafp*abs(f));

end

function phifn = phifn(f, deltafn)

    % Per (6) in Zhu, W. H., & Piedboeuf, J. C. (2005).
    phifn = f/(1 + deltafn*abs(f));

end

function phivp = phivp(v)

    % Chosen as constant. More details on pp. 211 of Zhu, W. H., & 
    % Piedboeuf, J. C. (2005), just above Eq. (71)
    phivp = 5 + 0*v;

end

function phivn = phivn(v)

    % Chosen as constant. More details on pp. 211 of Zhu, W. H., & 
    % Piedboeuf, J. C. (2005), just above Eq. (71)
    phivn = 5 + 0*v;

end

== matlab function VDCHyd2022a/sbCartesianControl/velocityJacobianFunction ==
  data: theta1 input; J output; theta2 input; xt2 input
function J = velocityJacobian(theta1, theta2, xt2)

    % Velocity Jacobian matrix in the present example, relating the TCP
    % velocity in the world frame with joint velocities.
    % W_V_D22 = J * q'
    % The derivation is provided in the supplementary pdf.
    J11 = -0.1*cos(theta1) - 0.152638*cos(theta1+theta2) - 1.59687*sin(theta1) + (-1.99949 - xt2)*sin(theta1 + theta2);
    J12 = -0.152638*cos(theta1 + theta2) + (-1.99949 - xt2)*sin(theta1 + theta2);
    J13 = cos(theta1 + theta2);
    J21 = cos(theta1)*(1.59687 + (1.99949 + xt2) * cos(theta2) - 0.154167*sin(theta2)) + sin(theta1)*(-0.1 - 0.154167*cos(theta2) + (-1.99949-xt2)*sin(theta2));
    J22 = cos(theta1)*((1.99949 + xt2)*cos(theta2) - 0.154167*sin(theta2)) + sin(theta1)*(-0.154167*cos(theta2) + (-1.99949 - xt2)*sin(theta2));
    J23 = cos(theta2)*sin(theta1) + cos(theta1)*sin(theta2);
    J = [J11 J12 J13; J21 J22 J23];

end

== matlab function VDCHyd2022a/sbVDCController/sbFormingControlActions/sbFrictionRegressorPS2/frictionRegressorFunctionPS2 ==
  data: v input; z input; Yf output; L input; Fd input; frictionPS2 parameter
function Yf = frictionRegressor(v,z,L, Fd, frictionPS2)

    % Forms the friction regressor from Zhu, W. H., & Piedboeuf, J. C. 
    % (2005). Adaptive output force tracking control of hydraulic cylinders 
    % with applications to robot manipulators.
    Yf = [(1 - L)*g(z, frictionPS2.zss)*S(z),...
          -(1 - L)*g(-z, frictionPS2.zss)*S(-z),...
          1 - L,...
          (1 - L)*S(v)*phivp(v)*v,...
          (1 - L)*S(-v)*phivn(v)*v,...
          S(Fd)*L*phifp(Fd,frictionPS2.deltap),...
          S(-Fd)*L*phifn(Fd,frictionPS2.deltan)];

end

function S = S(x)

    % Per (2) from Zhu, W. H., & Piedboeuf, J. C. (2005).
    if x > 0
        S = 1;
    else
        S = 0;
    end

end

function g = g(z, zss)

    % Per (5) in Zhu, W. H., & Piedboeuf, J. C. (2005).
    if z >= zss
        g = 1;
    elseif z <= 0
        g = 0;
    else
        g = z/zss;
    end

end

function phifp = phifp(f, deltafp)

    % Per (6) in Zhu, W. H., & Piedboeuf, J. C. (2005).
    phifp = f/(1 + deltafp*abs(f));

end

function phifn = phifn(f, deltafn)

    % Per (6) in Zhu, W. H., & Piedboeuf, J. C. (2005).
    phifn = f/(1 + deltafn*abs(f));

end

function phivp = phivp(v)

    % Chosen as constant. More details on pp. 211 of Zhu, W. H., & 
    % Piedboeuf, J. C. (2005), just above Eq. (71)
    phivp = 5 + 0*v;

end

function phivn = phivn(v)

    % Chosen as constant. More details on pp. 211 of Zhu, W. H., & 
    % Piedboeuf, J. C. (2005), just above Eq. (71)
    phivn = 5 + 0*v;

end

== matlab function VDCHyd2022a/sbVDCController/sbFormingControlActions/sbFrictionRegressorRS2/frictionRegressorFunctionRS2 ==
  data: v input; z input; Yf output; L input; Fd input; frictionRS2 parameter
function Yf = frictionRegressor(v,z,L, Fd, frictionRS2)

    % Forms the friction regressor from Zhu, W. H., & Piedboeuf, J. C. 
    % (2005). Adaptive output force tracking control of hydraulic cylinders 
    % with applications to robot manipulators.
    Yf = [(1 - L)*g(z, frictionRS2.zss)*S(z),...
          -(1 - L)*g(-z, frictionRS2.zss)*S(-z),...
          1 - L,...
          (1 - L)*S(v)*phivp(v)*v,...
          (1 - L)*S(-v)*phivn(v)*v,...
          S(Fd)*L*phifp(Fd,frictionRS2.deltap),...
          S(-Fd)*L*phifn(Fd,frictionRS2.deltan)];

end

function S = S(x)

    % Per (2) from Zhu, W. H., & Piedboeuf, J. C. (2005).
    if x > 0
        S = 1;
    else
        S = 0;
    end

end

function g = g(z, zss)

    % Per (5) in Zhu, W. H., & Piedboeuf, J. C. (2005).
    if z >= zss
        g = 1;
    elseif z <= 0
        g = 0;
    else
        g = z/zss;
    end

end

function phifp = phifp(f, deltafp)

    % Per (6) in Zhu, W. H., & Piedboeuf, J. C. (2005).
    phifp = f/(1 + deltafp*abs(f));

end

function phifn = phifn(f, deltafn)

    % Per (6) in Zhu, W. H., & Piedboeuf, J. C. (2005).
    phifn = f/(1 + deltafn*abs(f));

end

function phivp = phivp(v)

    % Chosen as constant. More details on pp. 211 of Zhu, W. H., & 
    % Piedboeuf, J. C. (2005), just above Eq. (71)
    phivp = 5 + 0*v;

end

function phivn = phivn(v)

    % Chosen as constant. More details on pp. 211 of Zhu, W. H., & 
    % Piedboeuf, J. C. (2005), just above Eq. (71)
    phivn = 5 + 0*v;

end

== matlab function VDCHyd2022a/sbVDCController/sbFormingControlActions/sbFrictionRegressorRS1/frictionRegressorFunctionRS1 ==
  data: v input; z input; Yf output; L input; Fd input; frictionRS1 parameter
function Yf = frictionRegressor(v,z,L, Fd, frictionRS1)

    % Forms the friction regressor from Zhu, W. H., & Piedboeuf, J. C. 
    % (2005). Adaptive output force tracking control of hydraulic cylinders 
    % with applications to robot manipulators.
    Yf = [(1 - L)*g(z, frictionRS1.zss)*S(z),...
          -(1 - L)*g(-z, frictionRS1.zss)*S(-z),...
          1 - L,...
          (1 - L)*S(v)*phivp(v)*v,...
          (1 - L)*S(-v)*phivn(v)*v,...
          S(Fd)*L*phifp(Fd,frictionRS1.deltap),...
          S(-Fd)*L*phifn(Fd,frictionRS1.deltan)];

end

function S = S(x)

    % Per (2) from Zhu, W. H., & Piedboeuf, J. C. (2005).
    if x > 0
        S = 1;
    else
        S = 0;
    end

end

function g = g(z, zss)

    % Per (5) in Zhu, W. H., & Piedboeuf, J. C. (2005).
    if z >= zss
        g = 1;
    elseif z <= 0
        g = 0;
    else
        g = z/zss;
    end

end

function phifp = phifp(f, deltafp)

    % Per (6) in Zhu, W. H., & Piedboeuf, J. C. (2005).
    phifp = f/(1 + deltafp*abs(f));

end

function phifn = phifn(f, deltafn)

    % Per (6) in Zhu, W. H., & Piedboeuf, J. C. (2005).
    phifn = f/(1 + deltafn*abs(f));

end

function phivp = phivp(v)

    % Chosen as constant. More details on pp. 211 of Zhu, W. H., & 
    % Piedboeuf, J. C. (2005), just above Eq. (71)
    phivp = 5 + 0*v;

end

function phivn = phivn(v)

    % Chosen as constant. More details on pp. 211 of Zhu, W. H., & 
    % Piedboeuf, J. C. (2005), just above Eq. (71)
    phivn = 5 + 0*v;

end

== matlab function VDCHyd2022a/sbHydraulicElements/sbValveFlowsRS1/liftValveFlows ==
  data: pa1 input; Qa1 output; pb1 input; u1v input; pS input; pR input; Qb1 output; valve1 parameter
function [Qa1, Qb1] = liftValveFlows(pa1, pb1, u1v, pS, pR, valve1)

    % Calculates lift valve flows per the paper equations (82) and (83).
    Qa1 = valve1.cp1*sqAbsPresDrop(pS - pa1)*u1v*selFcn(u1v) + ...
          valve1.cn1*sqAbsPresDrop(pa1 - pR)*u1v*selFcn(-u1v);
    Qb1 = -valve1.cn2*sqAbsPresDrop(pb1 - pR)*u1v*selFcn(u1v) - ...
          valve1.cp2*sqAbsPresDrop(pS - pb1)*u1v*selFcn(-u1v);
   
end

function S = selFcn(U)

    % Implements the selection function (84).
    if U > 0
        S = 1;
    else
        S = 0;
    end
    
end

function nup = sqAbsPresDrop(dp)

    % Implements the pressure drop function (85).
    nup = sign(dp)*sqrt(abs(dp));

end

== matlab function VDCHyd2022a/sbHydraulicElements/sbValveFlowsRS2/tiltValveFlows ==
  data: pa2 input; Qa2 output; pb2 input; u2v input; pS input; pR input; Qb2 output; valve2 parameter
function [Qa2, Qb2] = tiltValveFlows(pa2, pb2, u2v, pS, pR, valve2)

    % Calculates tilt valve flows per the paper equations (82) and (83).
    Qa2 = valve2.cp1*sqAbsPresDrop(pS - pa2)*u2v*selFcn(u2v) + ...
       valve2.cn1*sqAbsPresDrop(pa2 - pR)*u2v*selFcn(-u2v);
    Qb2 = -valve2.cn2*sqAbsPresDrop(pb2 - pR)*u2v*selFcn(u2v) - ...
       valve2.cp2*sqAbsPresDrop(pS - pb2)*u2v*selFcn(-u2v);
   
end

function S = selFcn(U)

    % Implements the selection function (84).    
    if U > 0
        S = 1;
    else
        S = 0;
    end
    
end

function nup = sqAbsPresDrop(dp)

    % Implements the pressure drop function (85).
    nup = sign(dp)*sqrt(abs(dp));

end
